simulink model "PMSLM_Close_Loop_MBDL4"  (R2026a)
settings: Solver=FixedStepDiscrete  StopTime=Inf  FixedStep=Ts  EnableMultiTasking=on
values from neighbouring files (symbols this model uses):
  ADC_GainA = 0.01664    [PMSLM_Init_Params_MBDL4.m]
  ADC_GainB = 0.01664    [PMSLM_Init_Params_MBDL4.m]
  ADC_GainC = 0.01664    [PMSLM_Init_Params_MBDL4.m]
  Close_Loop_EN = Simulink.Parameter    [PMSLM_Init_Params_MBDL4.m]
  CPU_Clock = 200e6    (= 200000000)    [PMSLM_Init_Params_MBDL4.m]    (also in init_PMLSM_ThreeLoop_Simple.m)
  delay_N = 50    [PMSLM_Init_Params_MBDL4.m]
  ENCON_Manual = Simulink.Parameter    [PMSLM_Init_Params_MBDL4.m]
  FReset_Manual = Simulink.Parameter    [PMSLM_Init_Params_MBDL4.m]
  GPIO30_PWM_OE_Disable = Simulink.Parameter    [PMSLM_Init_Params_MBDL4.m]
  Grating_Resolution_mm_per_count = 0.0001    [PMSLM_Init_Params_MBDL4.m]
  Hold_Ticks = 30000    [PMSLM_Init_Params_MBDL4.m]
  Id_Init_Step = Id_Init_Target / Ramp_Ticks    (= 5e-05)    [PMSLM_Init_Params_MBDL4.m]
  Id_Init_Target = 0.5    [PMSLM_Init_Params_MBDL4.m]
  Id_Ref_Set = Simulink.Parameter    [PMSLM_Init_Params_MBDL4.m]
  Init_Reset = Simulink.Parameter    [PMSLM_Init_Params_MBDL4.m]
  Init_Start = Simulink.Parameter    [PMSLM_Init_Params_MBDL4.m]
  Iq_fric_run = 0.05    [PMSLM_Init_Params_MBDL4.m]
  Iq_fric_start = 0.40    (= 0.4)    [PMSLM_Init_Params_MBDL4.m]
  Iq_int_limit = 0.10    (= 0.1)    [PMSLM_Init_Params_MBDL4.m]    (also in init_PMLSM_ThreeLoop_Simple.m = 0.5)
  Iq_Test_Mode = Simulink.Parameter    [PMSLM_Init_Params_MBDL4.m]
  Iq_Test_Ref = Simulink.Parameter    [PMSLM_Init_Params_MBDL4.m]
  Kaw_d = Kaw_q    (= 0.2)    [PMSLM_Init_Params_MBDL4.m]    (also in init_PMLSM_ThreeLoop_Simple.m = Tuning_Gains.Kaw_d)
  Kaw_q = 0.2    [PMSLM_Init_Params_MBDL4.m]    (also in init_PMLSM_ThreeLoop_Simple.m = Tuning_Gains.Kaw_q)
  Kaw_s = 0.4    [PMSLM_Init_Params_MBDL4.m]    (also in init_PMLSM_ThreeLoop_Simple.m = Tuning_Gains.Kaw_s)
  Ki_ACR = ACR_Commissioning_Scale*Ki_ACR_Baseline    (= 2962.5)    [PMSLM_Init_Params_MBDL4.m]    (also in init_PMLSM_ThreeLoop_Simple.m = Tuning_Gains.Ki_ACR; init_PMLSM_mil_test_params.m = Kp_ACR*PMLSM_Rs_ohm/PMLSM_Lq_H)
  Ki_ASR = 0.05    [PMSLM_Init_Params_MBDL4.m]    (also in init_PMLSM_ThreeLoop_Simple.m = Tuning_Gains.Ki_ASR)
  Kp_ACR = ACR_Commissioning_Scale*Kp_ACR_Baseline    (= 2.18125)    [PMSLM_Init_Params_MBDL4.m]    (also in init_PMLSM_ThreeLoop_Simple.m = Tuning_Gains.Kp_ACR; init_PMLSM_mil_test_params.m = PMLSM_Lq_H/(4*MIL_AUM3S4_Current_PI_xi^2*MIL_AUM3S4_Current_)
  Kp_ASR = 0.03    [PMSLM_Init_Params_MBDL4.m]    (also in init_PMLSM_ThreeLoop_Simple.m = Tuning_Gains.Kp_ASR)
  Kp_pos = 5    [PMSLM_Init_Params_MBDL4.m]    (also in init_PMLSM_ThreeLoop_Simple.m = Tuning_Gains.Kp_pos)
  OffsetCal_EN = Simulink.Parameter    [PMSLM_Init_Params_MBDL4.m]
  PI_Reset_EN = Simulink.Parameter    [PMSLM_Init_Params_MBDL4.m]
  PMLSM_Ld_H = Ld    (= 0.001745)    [PMSLM_Init_Params_MBDL4.m]    (also in init_PMLSM_ThreeLoop_Simple.m; init_PMLSM_plant_params.m)
  PMLSM_Lq_H = Lq    (= 0.001745)    [PMSLM_Init_Params_MBDL4.m]    (also in init_PMLSM_ThreeLoop_Simple.m; init_PMLSM_plant_params.m)
  PMLSM_psi_f_Wb = flux    (= 0.141)    [PMSLM_Init_Params_MBDL4.m]    (also in init_PMLSM_ThreeLoop_Simple.m; init_PMLSM_plant_params.m)
  Pos_deadband = 0.02    [PMSLM_Init_Params_MBDL4.m]    (also in init_PMLSM_ThreeLoop_Simple.m)
  Pos_Loop_EN = Simulink.Parameter    [PMSLM_Init_Params_MBDL4.m]
  qep_mid_cnt = 2147483648    [PMSLM_Init_Params_MBDL4.m]
  Ramp_Ticks = 10000    [PMSLM_Init_Params_MBDL4.m]
  RELCON_Manual = Simulink.Parameter    [PMSLM_Init_Params_MBDL4.m]
  Speed_loop_Iq_Limit = Iq_Limit    (= 0.3)    [PMSLM_Init_Params_MBDL4.m]    (also in init_PMLSM_ThreeLoop_Simple.m = 1)
  Tau_e_mm = 60    [PMSLM_Init_Params_MBDL4.m]
  theta_align_const = 0    [PMSLM_Init_Params_MBDL4.m]
  Theta_Offset_Fine = Simulink.Parameter    [PMSLM_Init_Params_MBDL4.m]
  Three_Current_Sampling_EN = Simulink.Parameter    [PMSLM_Init_Params_MBDL4.m]
  Ts = 1 / PWM_Freq    (= 0.0001)    [PMSLM_Init_Params_MBDL4.m]    (also in init_PMLSM_ThreeLoop_Simple.m)
  Ts_ACR = 1e-4    (= 0.0001)    [PMSLM_Init_Params_MBDL4.m]    (also in init_PMLSM_ThreeLoop_Simple.m)
  Ts_ASR = 1e-3    (= 0.001)    [PMSLM_Init_Params_MBDL4.m]    (also in init_PMLSM_ThreeLoop_Simple.m)
  Udc = 48    [PMSLM_Init_Params_MBDL4.m]    (also in init_PMLSM_ThreeLoop_Simple.m; init_PMLSM_mil_test_params.m)
  Uq_Zero_EN = 0：q 轴用正常 PI    [PMSLM_Init_Params_MBDL4.m]
  v_ff_eps = 0.5    [PMSLM_Init_Params_MBDL4.m]    (also in init_PMLSM_ThreeLoop_Simple.m)
  V_meas_max = 500    [PMSLM_Init_Params_MBDL4.m]
  v_meas_zero_eps = 0.5    [PMSLM_Init_Params_MBDL4.m]
  v_over_eps = 3    [PMSLM_Init_Params_MBDL4.m]    (also in init_PMLSM_ThreeLoop_Simple.m)
  V_pos_max_mmps = 10    [PMSLM_Init_Params_MBDL4.m]    (also in init_PMLSM_ThreeLoop_Simple.m = 20)
  v_ref_max = 20    [PMSLM_Init_Params_MBDL4.m]    (also in init_PMLSM_ThreeLoop_Simple.m)
  v_ref_set = Simulink.Parameter    [PMSLM_Init_Params_MBDL4.m]
  v_ref_set_step_dn = v_ref_set_rate_dn * Ts    (= 0.005)    [PMSLM_Init_Params_MBDL4.m]    (also in init_PMLSM_ThreeLoop_Simple.m)
  v_ref_set_step_up = v_ref_set_rate_up * Ts    (= 0.005)    [PMSLM_Init_Params_MBDL4.m]    (also in init_PMLSM_ThreeLoop_Simple.m)
  v_ref_zero_eps = 0.2    [PMSLM_Init_Params_MBDL4.m]    (also in init_PMLSM_ThreeLoop_Simple.m = 0)
  v_stick_off = 3.0    (= 3)    [PMSLM_Init_Params_MBDL4.m]
  v_stick_on = 1.0    (= 1)    [PMSLM_Init_Params_MBDL4.m]
  X_max_hard = 500    [PMSLM_Init_Params_MBDL4.m]
  X_max_soft = 470    [PMSLM_Init_Params_MBDL4.m]
  X_min_hard = -500    [PMSLM_Init_Params_MBDL4.m]
  X_min_soft = -470    [PMSLM_Init_Params_MBDL4.m]
  x_ref_mm = Simulink.Parameter    [PMSLM_Init_Params_MBDL4.m]
undefined symbols (not defined in the file or in its folder): bit, Down, GPTRIP1SEL, TZ1, Up
libraries: simulink x11, c2802xlib x6, c2838xlib x6, mcbeeMathTransformLib x2, c280xlib x1, mcbcontrolslib x1, svdschedulerlib x1
(part 1 of 2)
settings Model: ExtModeTrigDuration=8  Creator=lww  LastModifiedBy=lww
settings OptimizationCC: DefaultUnderspecifiedDataType=single  MaxStackSize=1024
settings DebuggingCC: ArtificialAlgebraicLoopMsg=none
settings HardwareCC: ProdBitPerChar=16.0  ProdBitPerInt=16.0  ProdLargestAtomicInteger=Integer  ProdWordSize=16.0  ProdHWDeviceType=Texas Instruments->C2000  HardwareBoardFeatureSet=SoCBlockset
settings ModelReferenceCC: ModelReferenceNumInstancesAllowed=Single
settings RTWCC: SystemTargetFile=ert.tlc  HardwareBoard=TI F2838x  TLCOptions=-aInlineSetEventsForThisBaseRateFcn=TLC_FALSE -aSuppressMultiTaskScheduler=TLC_FALSE -aRateBasedStepFcn=1  Toolchain=Texas Instruments Code Composer Studio - EABI (C2000)  CodeProfilingSaveOptions=MetricsOnly  Description=Embedded Coder
settings ERTTargetCC: ExtModeTransport=4.0  ExtModeAutomaticAllocSize=off  ExtModeStaticAllocSize=10000.0  DynamicArrayContainerType=coder::array  CodeReplacementLibrary=TI C28x  SubcomponentCodeInterfacePackaging=Nonreusable function
settings SimscapeCC: SimscapeNominalValues="[{\"value\":\"1\",\"unit\":\"A\"},{\"value\":\"1\",\"unit\":\"bar\"},{\"value\":\"1\",\"unit\":\"cm^2\"},{\"value\":\"1\",\"unit\":\"cm^3/s\"},{\"value\":\"1\",\"unit\":\"kJ/kg\"},{\"value\":\"1\",\"unit\":\"kW\"},{\"value\":\"1\",\"unit\":\"l\"},{\"value\":\"1\",\"unit\":\"N\"},{\"value\":\"1\",\"unit\":\"N*m\"},{\"value\":\"1\",\"unit\":\"V\"}]"  SimscapeLogType=none  SimscapeLogDataHistory=5000.0

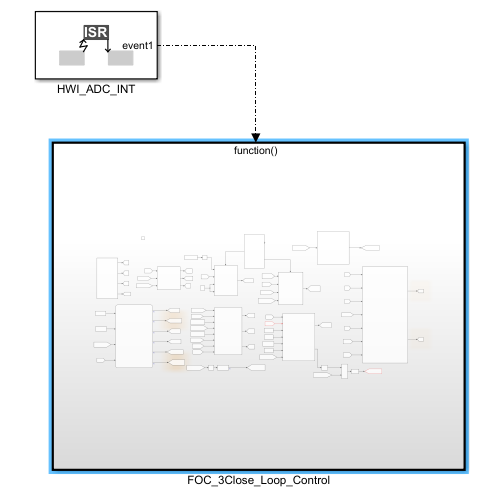
[thumbnail: Simulink's stored preview of the top-level diagram]
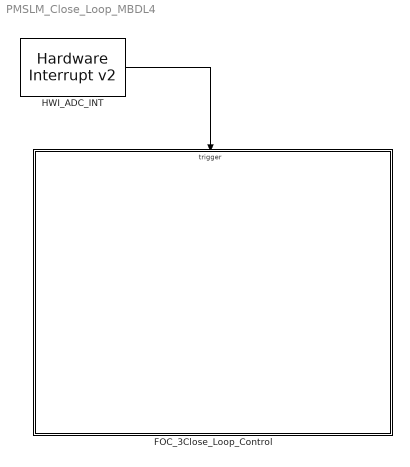
== system PMSLM_Close_Loop_MBDL4 ==
  FOC_3Close_Loop_Control : Subsystem  TreatAsAtomicUnit=on
  HWI_ADC_INT : svdschedulerlib/Hardware Interrupt v2  ISRGroup=ADC - Analog to Digital Converter  ISRName=ADCA1_INT  ISRNumber=32  NumEventsToServe=1  EventsList={'on','EOC event','1';'off','Overflow event','2';'off','Custom event','3'}  SelectedEvents={'event1'}  TaskPriority=30  DisablePreemption=on  ClearInterruptFlagsAtEndOfEvent=on  InterruptDefinitionFile=$(TARGET_ROOT)/registry/interrupts/TIF2838x_c28xCPU1_interrupts.xml  HardwareBoard=TI F2838x  EnableSimPort=off
  wires:
  HWI_ADC_INT/1 -> FOC_3Close_Loop_Control/Trigger

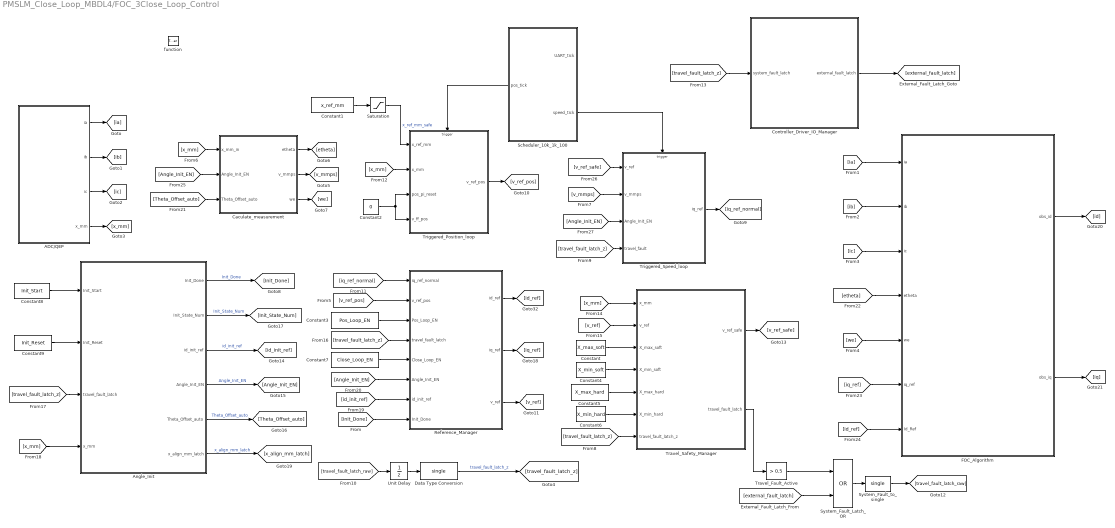
== system PMSLM_Close_Loop_MBDL4/FOC_3Close_Loop_Control ==
  function : TriggerPort  TriggerType=function-call  VariantControl=(inherit)
  ADC/QEP : Subsystem
  Angle_Init : Stateflow chart  TreatAsAtomicUnit=on
  Caculate_measurement : Subsystem
  Constant : Constant  Value=X_max_soft
  Constant1 : Constant  Value=x_ref_mm
  Constant2 : Constant  Value=0
  Constant3 : Constant  Value=Pos_Loop_EN
  Constant4 : Constant  Value=X_min_soft
  Constant5 : Constant  Value=X_max_hard
  Constant6 : Constant  Value=X_min_hard
  Constant7 : Constant  Value=Close_Loop_EN
  Constant8 : Constant  Value=Init_Start
  Constant9 : Constant  Value=Init_Reset
  Controller_Driver_IO_Manager : Subsystem
  Data Type Conversion : DataTypeConversion  OutDataTypeStr=single  SaturateOnIntegerOverflow=off  RndMeth=Floor
  FOC_Algorithm : Subsystem
  Reference_Manager : Subsystem
  Saturation : Saturate  UpperLimit=X_max_soft  LowerLimit=X_min_soft
  Scheduler_10k_1k_100 : Subsystem
      settings: PortSchema="{\"entries\":[{\"content\":{\"sides\":[{\"content\":{\"connectorIds\":[\"Out3\"]},\"type\":\"ConnectorPlacement.EquallySpacedRectSide\",\"uuid\":\"7a2cd2ad-1b6d-4ced-b4c0-dea2e76e4441\"},{\"content\":{\"connectorIds\":[\"Out1\",\"Out2\"],\"side\":\"RIGHT\"},\"type\":\"ConnectorPlacement.EquallySpacedRectSide\",\"uuid\":\"f7db3b94-1126-4089-83bd-8e57d20e6fd7\"},{\"content\":{\"side\":\"TOP\"},\"type\":\"ConnectorPlacement.EquallySpacedRectSide\",\"uuid\":\"9153f6b5-22af-48be-92c0-68be43f93648\"}]},\"type\":\"ConnectorPlacement.EquallySpacedConnector\",\"uuid\":\"029fb485-bddc-4cd2-9c64-7547c8dffd2b\"}],\"packageUris\":[\"http://schema.mathworks.com/mf0/Connector/R2020b\"],\"version\":\"1.0\"}"
  System_Fault_Latch_OR : Logic  Operator=OR
  System_Fault_to_single : DataTypeConversion  OutDataTypeStr=single
  Travel_Fault_Active : simulink/Logic and Bit Operations/Compare To Constant  relop=>  const=0.5  OutDataTypeStr=boolean
  Travel_Safety_Manager : MATLAB Function  TreatAsAtomicUnit=on
  Triggered_Position_loop : Subsystem  TreatAsAtomicUnit=on
  Triggered_Speed_loop : Subsystem  TreatAsAtomicUnit=on
  Unit Delay : UnitDelay  SampleTime=-1
  wires:
  [iq_ref_normal] -> Reference_Manager/1(iq_ref_normal)
  ADC/QEP/3(ic) -> [ic]
  Caculate_measurement/2(v_mmps) -> [v_mmps]
  [v_mmps] -> Triggered_Speed_loop/2(v_mmps)
  Caculate_measurement/1(etheta) -> [etheta]
  Reference_Manager/1(id_ref) -> [id_ref]
  Scheduler_10k_1k_100/2(speed_tick) -> Triggered_Speed_loop/Trigger
  [v_ref_safe] -> Triggered_Speed_loop/1(v_ref)
  Reference_Manager/2(iq_ref) -> [iq_ref]
  ADC/QEP/1(ia) -> [ia]
  Triggered_Speed_loop/1(iq_ref) -> [iq_ref_normal]
  ADC/QEP/2(ib) -> [ib]
  [ia] -> FOC_Algorithm/1(ia)
  [ib] -> FOC_Algorithm/2(ib)
  [ic] -> FOC_Algorithm/3(ic)
  [etheta] -> FOC_Algorithm/4(etheta)
  [we] -> FOC_Algorithm/5(we)
  [iq_ref] -> FOC_Algorithm/6(iq_ref)
  [x_mm] -> Triggered_Position_loop/2(x_mm)
  Constant2/1 -> Triggered_Position_loop/3(pos_pi_reset), Triggered_Position_loop/4(v_ff_pos)
  Triggered_Position_loop/1(v_ref_pos) -> [v_ref_pos]
  [v_ref_pos] -> Reference_Manager/2(v_ref_pos)
  Constant3/1 -> Reference_Manager/3(Pos_Loop_EN)
  ADC/QEP/4(x_mm) -> [x_mm]
  Caculate_measurement/3(we) -> [we]
  [x_mm] -> Caculate_measurement/1(x_mm_in)
  Reference_Manager/3(v_ref) -> [v_ref]
  Constant1/1 -> Saturation/1
  Saturation/1 -> Triggered_Position_loop/1(x_ref_mm)  "x_ref_mm_safe"
  [travel_fault_latch_z] -> Triggered_Speed_loop/4(travel_fault)
  [travel_fault_latch_raw] -> Unit Delay/1
  [id_ref] -> FOC_Algorithm/7(Id_Ref)
  [travel_fault_latch_z] -> Controller_Driver_IO_Manager/1(system_fault_latch)
  [x_mm] -> Travel_Safety_Manager/1(x_mm)
  [v_ref] -> Travel_Safety_Manager/2(v_ref)
  Constant/1 -> Travel_Safety_Manager/3(X_max_soft)
  Constant4/1 -> Travel_Safety_Manager/4(X_min_soft)
  Constant5/1 -> Travel_Safety_Manager/5(X_max_hard)
  Constant6/1 -> Travel_Safety_Manager/6(X_min_hard)
  Travel_Safety_Manager/1(v_ref_safe) -> [v_ref_safe]
  [travel_fault_latch_z] -> Travel_Safety_Manager/7(travel_fault_latch_z)
  Unit Delay/1 -> Data Type Conversion/1
  Data Type Conversion/1 -> [travel_fault_latch_z]  "travel_fault_latch_z"
  [travel_fault_latch_z] -> Reference_Manager/4(travel_fault_latch)
  Constant7/1 -> Reference_Manager/5(Close_Loop_EN)
  Constant8/1 -> Angle_Init/1(Init_Start)
  Constant9/1 -> Angle_Init/2(Init_Reset)
  [travel_fault_latch_z] -> Angle_Init/3(travel_fault_latch)
  Angle_Init/1(Init_Done) -> [Init_Done]  "Init_Done"
  [Init_Done] -> Reference_Manager/8(Init_Done)
  [x_mm] -> Angle_Init/4(x_mm)
  Angle_Init/3(id_init_ref) -> [id_init_ref]  "id_init_ref"
  [id_init_ref] -> Reference_Manager/7(id_init_ref)
  Angle_Init/4(Angle_Init_EN) -> [Angle_Init_EN]  "Angle_Init_EN"
  [Angle_Init_EN] -> Reference_Manager/6(Angle_Init_EN)
  Angle_Init/5(Theta_Offset_auto) -> [Theta_Offset_auto]  "Theta_Offset_auto"
  [Theta_Offset_auto] -> Caculate_measurement/3(Theta_Offset_auto)
  [Angle_Init_EN] -> Caculate_measurement/2(Angle_Init_EN)
  Angle_Init/2(Init_State_Num) -> [Init_State_Num]  "Init_State_Num"
  [Angle_Init_EN] -> Triggered_Speed_loop/3(Angle_Init_EN)
  Angle_Init/6(x_align_mm_latch) -> [x_align_mm_latch]  "x_align_mm_latch"
  FOC_Algorithm/1(obs_id) -> [id]
  FOC_Algorithm/2(obs_iq) -> [iq]
  Scheduler_10k_1k_100/3(pos_tick) -> Triggered_Position_loop/Trigger
  Travel_Safety_Manager/2(travel_fault_latch) -> Travel_Fault_Active/1
  Travel_Fault_Active/1 -> System_Fault_Latch_OR/1
  System_Fault_Latch_OR/1 -> System_Fault_to_single/1
  System_Fault_to_single/1 -> [travel_fault_latch_raw]
  Controller_Driver_IO_Manager/1(external_fault_latch) -> [external_fault_latch]
  [external_fault_latch] -> System_Fault_Latch_OR/2

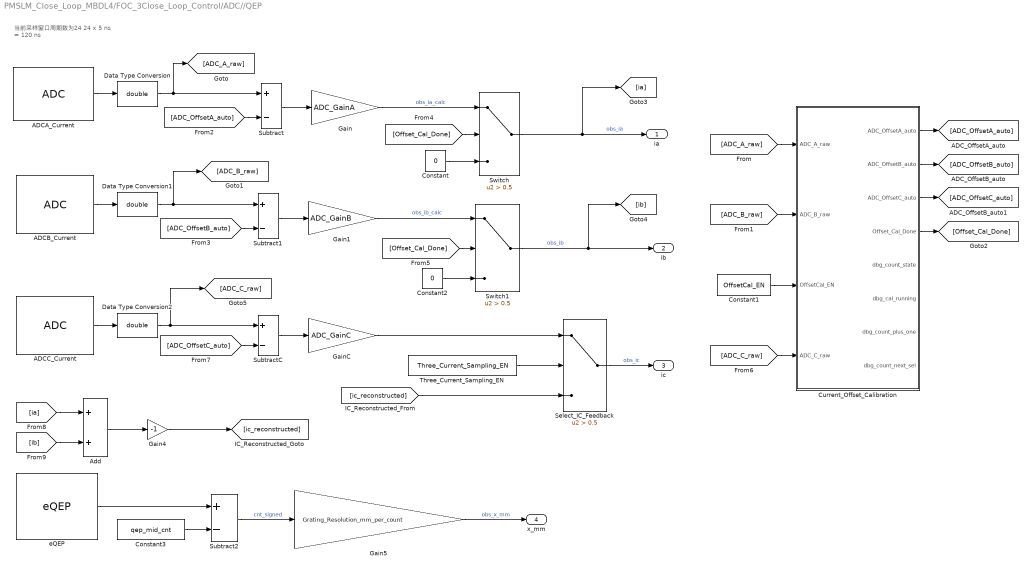
== system PMSLM_Close_Loop_MBDL4/FOC_3Close_Loop_Control/ADC//QEP ==
  note: 当前采样窗口周期数为24
      | 24 x 5 ns = 120 ns
  ADCA_Current : c2802xlib/ADC  blkParamProc=C2000_Type4  ADCModule=A  samplingMode=Single sample mode  ADCResolution=12-bit (Single-ended input)  ADC29xResolution=12-bit  ADCMode=Single-ended input  useSOC1=SOC0  useSOC2=SOC0_SOC1  SOCAcquisitionWindow=24  SOCTriggerSource=ePWM1_ADCSOCA  SOCInterruptTrigger=No ADCINT  Ts=-1  dType=uint16  postInterrupt=on  interruptSel=ADCINT1  ADCINTContinuous=off  endma=off  chdma=1  conv1=ADCINA0  conv2=ADCINA0 and ADCINB0  conv1_Type4=ADCIN0  conv2_Type4=ADCIN0 and ADCIN1
      settings: LibrarySourceBlock=c2838xlib/ADC
  ADCB_Current : c2802xlib/ADC  blkParamProc=C2000_Type4  ADCModule=B  samplingMode=Single sample mode  ADCResolution=12-bit (Single-ended input)  ADC29xResolution=12-bit  ADCMode=Single-ended input  useSOC1=SOC0  useSOC2=SOC0_SOC1  SOCAcquisitionWindow=24  SOCTriggerSource=ePWM1_ADCSOCA  SOCInterruptTrigger=No ADCINT  Ts=-1  dType=uint16  postInterrupt=off  interruptSel=ADCINT1  ADCINTContinuous=on  endma=off  chdma=1  conv1=ADCINA0  conv2=ADCINA0 and ADCINB0  conv1_Type4=ADCIN0  conv2_Type4=ADCIN0 and ADCIN1
      settings: LibrarySourceBlock=c2838xlib/ADC
  ADCC_Current : c2802xlib/ADC  blkParamProc=C2000_Type4  ADCModule=C  samplingMode=Single sample mode  ADCResolution=12-bit (Single-ended input)  ADC29xResolution=12-bit  ADCMode=Single-ended input  useSOC1=SOC0  useSOC2=SOC0_SOC1  SOCAcquisitionWindow=24  SOCTriggerSource=ePWM1_ADCSOCA  SOCInterruptTrigger=No ADCINT  Ts=-1  dType=uint16  postInterrupt=off  interruptSel=ADCINT1  ADCINTContinuous=on  endma=off  chdma=1  conv1=ADCINA0  conv2=ADCINA0 and ADCINB0  conv1_Type4=ADCIN2  conv2_Type4=ADCIN0 and ADCIN1
      settings: LibrarySourceBlock=c2838xlib/ADC
  Add : Sum
  Constant : Constant  Value=0  OutDataTypeStr=double
  Constant1 : Constant  Value=OffsetCal_EN
  Constant2 : Constant  Value=0  OutDataTypeStr=double
  Constant3 : Constant  Value=qep_mid_cnt
  Current_Offset_Calibration : Subsystem
  Data Type Conversion : DataTypeConversion  OutDataTypeStr=double  SaturateOnIntegerOverflow=off  RndMeth=Floor
  Data Type Conversion1 : DataTypeConversion  OutDataTypeStr=double  SaturateOnIntegerOverflow=off  RndMeth=Floor
  Data Type Conversion2 : DataTypeConversion  OutDataTypeStr=double
  Gain : Gain  Gain=ADC_GainA
  Gain1 : Gain  Gain=ADC_GainB
  Gain4 : Gain  Gain=-1  OutDataTypeStr=double
  Gain5 : Gain  Gain=Grating_Resolution_mm_per_count
  GainC : Gain  Gain=ADC_GainC
  Select_IC_Feedback : Switch  Criteria=u2 > Threshold  Threshold=0.5  OutDataTypeStr=double
  Subtract : Sum  Inputs=+-
  Subtract1 : Sum  Inputs=+-
  Subtract2 : Sum  Inputs=+-
  SubtractC : Sum  Inputs=+-
  Switch : Switch  Criteria=u2 > Threshold  Threshold=0.5  OutDataTypeStr=double  SaturateOnIntegerOverflow=off  InputSameDT=off
  Switch1 : Switch  Criteria=u2 > Threshold  Threshold=0.5  OutDataTypeStr=double  SaturateOnIntegerOverflow=off  InputSameDT=off
  Three_Current_Sampling_EN : Constant  Value=Three_Current_Sampling_EN
  eQEP : c280xlib/eQEP  useModule=eQEP1  pcInputmode=Quadrature-count  externalClockrate=2x resolution: Count the rising/falling edge  swapPolarityselection=Clockwise  qdfOutputport=off  qapPolarityselection=off  qbpPolarityselection=off  qipPolarityselection=off  qspPolarityselection=off  igatePolarityselection=off  sampleTime=-1  pcOutputport=on  pcMaximumvalue=4294967295  indexInitializationcheck=off  indexInitializationevent=Rising edge  strobeInitializationcheck=off  strobeInitializationevent=Rising edge  softwareInitializationcheck=off  softwareInitializationsource=Set to init value at start up  softwareInitializationmode=on  pcInitialvalue=qep_mid_cnt  pcResetmode=Reset on an index event  ieloutputport=off  indexEventlatch=Rising edge  seloutputport=off  strobeEventlatch=Rising edge  pcefOutputport=off  enableEqepcapture=off  qctmrOutputport=off  qcprdOutputport=off  captureTimerprescaler=128  upEventprescaler=128  overflowErrorflag=off  directionErrorflag=off  captureTimerposition=On position counter read  unitTimerperiod=100000000  captureTimerlatch=off  capturePeriodlatch=off  positionCounterlatch=off  soenPolarityselection=off  spselPolarityselection=Index pin is used for sync output  compareValuesource=Specify via dialog  shadowMode=Load on QPOSCNT=0  compareValue=4294967295  syncOutputwidth=1  polaritySyncoutput=Active high  watchdogEnable=off  watchdogTimer=65535  outport1Datatype=auto  outport2Datatype=auto  outport3Datatype=auto  outport4Datatype=auto  outport5Datatype=auto  outport6Datatype=auto  outport7Datatype=auto  outport8Datatype=auto  outport9Datatype=auto  outport10Datatype=auto  outport11Datatype=auto  outport12Datatype=auto  eqepinterrupt_pce=off  eqepinterrupt_qpe=off  eqepinterrupt_qdc=off  eqepinterrupt_wto=off  eqepinterrupt_pcu=off  eqepinterrupt_pco=off  eqepinterrupt_pcr=off  eqepinterrupt_pcm=off  eqepinterrupt_sel=off  eqepinterrupt_iel=off  eqepinterrupt_uto=off  pheOutputport=off  watchdogOutputport=off  outport13Datatype=auto  outport14Datatype=auto
      settings: LibrarySourceBlock=c2838xlib/eQEP
  ia : Outport
  ib : Outport  Port=2
  ic : Outport  Port=3
  x_mm : Outport  Port=4
  wires:
  ADCA_Current/1 -> Data Type Conversion/1
  Data Type Conversion/1 -> [ADC_A_raw], Subtract/1
  [ADC_OffsetA_auto] -> Subtract/2
  Subtract/1 -> Gain/1
  Gain/1 -> Switch/1  "obs_ia_calc"
  [Offset_Cal_Done] -> Switch/2
  Constant/1 -> Switch/3
  Switch/1 -> ia/1, [ia]  "obs_ia"
  ADCB_Current/1 -> Data Type Conversion1/1
  Data Type Conversion1/1 -> [ADC_B_raw], Subtract1/1
  [ADC_OffsetB_auto] -> Subtract1/2
  Subtract1/1 -> Gain1/1
  Gain1/1 -> Switch1/1  "obs_ib_calc"
  [Offset_Cal_Done] -> Switch1/2
  Constant2/1 -> Switch1/3
  Switch1/1 -> [ib], ib/1  "obs_ib"
  ADCC_Current/1 -> Data Type Conversion2/1
  Data Type Conversion2/1 -> [ADC_C_raw], SubtractC/1
  [ADC_OffsetC_auto] -> SubtractC/2
  SubtractC/1 -> GainC/1
  GainC/1 -> Select_IC_Feedback/1
  Three_Current_Sampling_EN/1 -> Select_IC_Feedback/2
  Select_IC_Feedback/1 -> ic/1  "obs_ic"
  [ia] -> Add/1
  [ib] -> Add/2
  Add/1 -> Gain4/1
  Gain4/1 -> [ic_reconstructed]
  eQEP/1 -> Subtract2/1
  Constant3/1 -> Subtract2/2
  Subtract2/1 -> Gain5/1  "cnt_signed"
  Gain5/1 -> x_mm/1  "obs_x_mm"
  [ADC_A_raw] -> Current_Offset_Calibration/1(ADC_A_raw)
  [ADC_B_raw] -> Current_Offset_Calibration/2(ADC_B_raw)
  Constant1/1 -> Current_Offset_Calibration/3(OffsetCal_EN)
  Current_Offset_Calibration/1(ADC_OffsetA_auto) -> [ADC_OffsetA_auto]
  Current_Offset_Calibration/2(ADC_OffsetB_auto) -> [ADC_OffsetB_auto]
  Current_Offset_Calibration/4(Offset_Cal_Done) -> [Offset_Cal_Done]
  [ic_reconstructed] -> Select_IC_Feedback/3
  [ADC_C_raw] -> Current_Offset_Calibration/4(ADC_C_raw)
  Current_Offset_Calibration/3(ADC_OffsetC_auto) -> [ADC_OffsetC_auto]

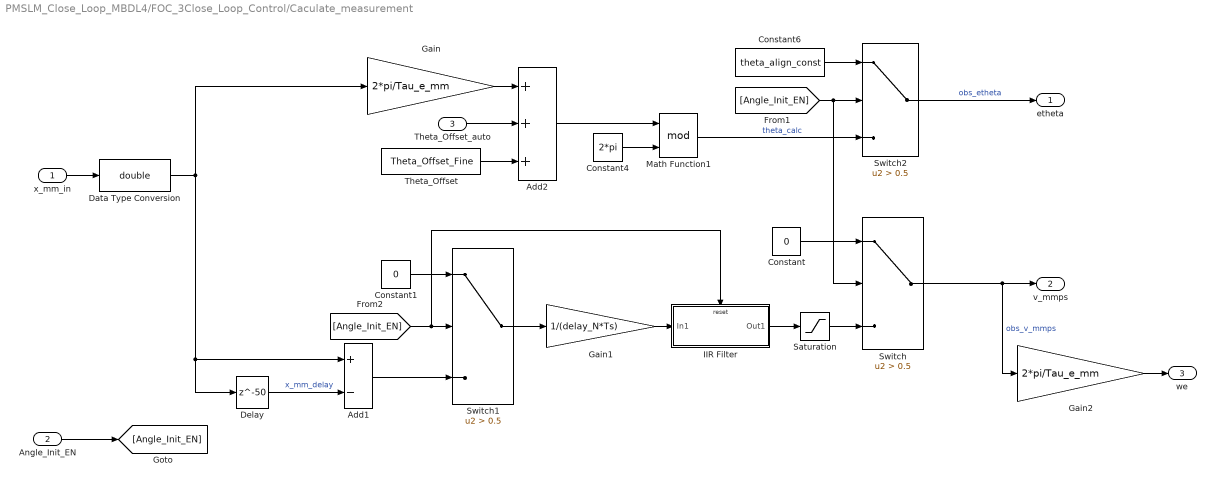
== system PMSLM_Close_Loop_MBDL4/FOC_3Close_Loop_Control/Caculate_measurement ==
  x_mm_in : Inport
  Angle_Init_EN : Inport  Port=2
  Theta_Offset_auto : Inport  Port=3
  Add1 : Sum  Inputs=+-
  Add2 : Sum  Inputs=+++
  Constant : Constant  Value=0
  Constant1 : Constant  Value=0
  Constant4 : Constant  Value=2*pi
  Constant6 : Constant  Value=theta_align_const
  Data Type Conversion : DataTypeConversion  OutDataTypeStr=double  SaturateOnIntegerOverflow=off  RndMeth=Floor
  Delay : Delay  DelayLength=50
  Gain : Gain  Gain=2*pi/Tau_e_mm
  Gain1 : Gain  Gain=1/(delay_N*Ts)
  Gain2 : Gain  Gain=2*pi/Tau_e_mm
  IIR Filter : Subsystem  TreatAsAtomicUnit=on
  Math Function1 : Math  Operator=mod
  Saturation : Saturate  UpperLimit=V_meas_max  LowerLimit=-V_meas_max
  Switch : Switch  Criteria=u2 > Threshold  Threshold=0.5  SaturateOnIntegerOverflow=off  InputSameDT=off
  Switch1 : Switch  Criteria=u2 > Threshold  Threshold=0.5  SaturateOnIntegerOverflow=off  InputSameDT=off
  Switch2 : Switch  Criteria=u2 > Threshold  Threshold=0.5  SaturateOnIntegerOverflow=off  InputSameDT=off
  Theta_Offset : Constant  Value=Theta_Offset_Fine
  etheta : Outport
  v_mmps : Outport  Port=2
  we : Outport  Port=3
  wires:
  x_mm_in/1 -> Data Type Conversion/1
  Delay/1 -> Add1/2  "x_mm_delay"
  Gain/1 -> Add2/1
  Add2/1 -> Math Function1/1
  Constant4/1 -> Math Function1/2
  Data Type Conversion/1 -> Delay/1, Add1/1, Gain/1
  Switch/1 -> Gain2/1, v_mmps/1  "obs_v_mmps"
  Constant/1 -> Switch/1
  Constant1/1 -> Switch1/1
  Switch1/1 -> Gain1/1
  Add1/1 -> Switch1/3
  IIR Filter/1(Out1) -> Saturation/1
  Gain1/1 -> IIR Filter/1(In1)
  Saturation/1 -> Switch/3
  [Angle_Init_EN] -> Switch2/2, Switch/2
  Math Function1/1 -> Switch2/3  "theta_calc"
  Switch2/1 -> etheta/1  "obs_etheta"
  Angle_Init_EN/1 -> [Angle_Init_EN]
  Constant6/1 -> Switch2/1
  Gain2/1 -> we/1
  [Angle_Init_EN] -> Switch1/2, IIR Filter/Reset
  Theta_Offset/1 -> Add2/3
  Theta_Offset_auto/1 -> Add2/2

== system PMSLM_Close_Loop_MBDL4/FOC_3Close_Loop_Control/Controller_Driver_IO_Manager ==
  note: GPIO30 only controls the PWM level-shifter active-low /OE.
      | RELCON, ENCON and F_Reset use independent GPIO outputs.
      | System fault: TZ1/TZ2 hardware trip + software latch; GPIO30=1 and RELCON/ENCON=0.
  note: GPIO67: ERRI; GPIO68: ERRU (active-low inputs)
  note: GPIO62: RELCON
  note: GPIO63: ENCON
  note: GPIO66: F_Reset
  note: GPIO30: PWM level-shifter /OE (1=disable, 0=enable)
  system_fault_latch : Inport
  Constant : Constant  Value=RELCON_Manual
  Constant2 : Constant  Value=GPIO30_PWM_OE_Disable
  Constant4 : Constant  Value=ENCON_Manual
  Constant5 : Constant  Value=FReset_Manual
  ENCON_Safe_Enable : Logic
  External_Fault_Latch : Subsystem
  GPIO30_PWM_OE : c2838xlib/Digital Output  GPIO_Number=GPIO24~GPIO31  GPIO_Bit0=off  GPIO_BIT0_Toggle=off  GPIO_Bit1=off  GPIO_BIT1_Toggle=off  GPIO_Bit2=off  GPIO_BIT2_Toggle=off  GPIO_Bit3=off  GPIO_BIT3_Toggle=off  GPIO_Bit4=off  GPIO_BIT4_Toggle=off  GPIO_Bit5=off  GPIO_BIT5_Toggle=off  GPIO_Bit6=on  GPIO_BIT6_Toggle=off  GPIO_Bit7=off  GPIO_BIT7_Toggle=off
  GPIO62_RELCON : c2838xlib/Digital Output  GPIO_Number=GPIO56~GPIO63  GPIO_Bit0=off  GPIO_BIT0_Toggle=off  GPIO_Bit1=off  GPIO_BIT1_Toggle=off  GPIO_Bit2=off  GPIO_BIT2_Toggle=off  GPIO_Bit3=off  GPIO_BIT3_Toggle=off  GPIO_Bit4=off  GPIO_BIT4_Toggle=off  GPIO_Bit5=off  GPIO_BIT5_Toggle=off  GPIO_Bit6=on  GPIO_BIT6_Toggle=off  GPIO_Bit7=off  GPIO_BIT7_Toggle=off
  GPIO63_ENCON : c2838xlib/Digital Output  GPIO_Number=GPIO56~GPIO63  GPIO_Bit0=off  GPIO_BIT0_Toggle=off  GPIO_Bit1=off  GPIO_BIT1_Toggle=off  GPIO_Bit2=off  GPIO_BIT2_Toggle=off  GPIO_Bit3=off  GPIO_BIT3_Toggle=off  GPIO_Bit4=off  GPIO_BIT4_Toggle=off  GPIO_Bit5=off  GPIO_BIT5_Toggle=off  GPIO_Bit6=off  GPIO_BIT6_Toggle=off  GPIO_Bit7=on  GPIO_BIT7_Toggle=off
  GPIO66_F_Reset : c2838xlib/Digital Output  GPIO_Number=GPIO64~GPIO71  GPIO_Bit0=off  GPIO_BIT0_Toggle=off  GPIO_Bit1=off  GPIO_BIT1_Toggle=off  GPIO_Bit2=on  GPIO_BIT2_Toggle=off  GPIO_Bit3=off  GPIO_BIT3_Toggle=off  GPIO_Bit4=off  GPIO_BIT4_Toggle=off  GPIO_Bit5=off  GPIO_BIT5_Toggle=off  GPIO_Bit6=off  GPIO_BIT6_Toggle=off  GPIO_Bit7=off  GPIO_BIT7_Toggle=off
  GPIO67_ERRI : c2838xlib/Digital Input  GPIO_Number=GPIO64~GPIO71  GPIO_Bit0=off  GPIO_Bit1=off  GPIO_Bit2=off  GPIO_Bit3=on  GPIO_Bit4=off  GPIO_Bit5=off  GPIO_Bit6=off  GPIO_Bit7=off  sampleTime=-1  dataType=boolean  GPIO_Bit0_Qualification=Sync to SYSCLKOUT  GPIO_Bit1_Qualification=Sync to SYSCLKOUT  GPIO_Bit2_Qualification=Sync to SYSCLKOUT  GPIO_Bit3_Qualification=Sync to SYSCLKOUT  GPIO_Bit4_Qualification=Sync to SYSCLKOUT  GPIO_Bit5_Qualification=Sync to SYSCLKOUT  GPIO_Bit6_Qualification=Sync to SYSCLKOUT  GPIO_Bit7_Qualification=Sync to SYSCLKOUT  Qualification_Period=-1
  GPIO68_ERRU : c2838xlib/Digital Input  GPIO_Number=GPIO64~GPIO71  GPIO_Bit0=off  GPIO_Bit1=off  GPIO_Bit2=off  GPIO_Bit3=off  GPIO_Bit4=on  GPIO_Bit5=off  GPIO_Bit6=off  GPIO_Bit7=off  sampleTime=-1  dataType=boolean  GPIO_Bit0_Qualification=Sync to SYSCLKOUT  GPIO_Bit1_Qualification=Sync to SYSCLKOUT  GPIO_Bit2_Qualification=Sync to SYSCLKOUT  GPIO_Bit3_Qualification=Sync to SYSCLKOUT  GPIO_Bit4_Qualification=Sync to SYSCLKOUT  GPIO_Bit5_Qualification=Sync to SYSCLKOUT  GPIO_Bit6_Qualification=Sync to SYSCLKOUT  GPIO_Bit7_Qualification=Sync to SYSCLKOUT  Qualification_Period=-1
  Logical Operator : Logic  Operator=OR  AllPortsSameDT=off  OutDataTypeStr=boolean
  RELCON_Safe_Enable : Logic
  System_Fault_Active : simulink/Logic and Bit Operations/Compare To Constant  relop=>  const=0.5  OutDataTypeStr=boolean
  System_Fault_Not : Logic  Operator=NOT  Inputs=1
  external_fault_latch : Outport  OutDataTypeStr=boolean  PortDimensions=1
  wires:
  Constant2/1 -> Logical Operator/1
  Logical Operator/1 -> GPIO30_PWM_OE/1
  system_fault_latch/1 -> System_Fault_Active/1
  System_Fault_Active/1 -> Logical Operator/2, System_Fault_Not/1
  System_Fault_Not/1 -> [drive_safe]
  GPIO67_ERRI/1 -> [ERRI_raw]
  [ERRI_raw] -> External_Fault_Latch/1(ERRI_raw)
  GPIO68_ERRU/1 -> [ERRU_raw]
  [ERRU_raw] -> External_Fault_Latch/2(ERRU_raw)
  Constant/1 -> RELCON_Safe_Enable/1  "obs_RELCON"
  RELCON_Safe_Enable/1 -> GPIO62_RELCON/1
  Constant4/1 -> ENCON_Safe_Enable/1
  [drive_safe] -> ENCON_Safe_Enable/2
  ENCON_Safe_Enable/1 -> GPIO63_ENCON/1
  Constant5/1 -> GPIO66_F_Reset/1
  External_Fault_Latch/1(external_fault_latch) -> external_fault_latch/1
  [drive_safe] -> RELCON_Safe_Enable/2

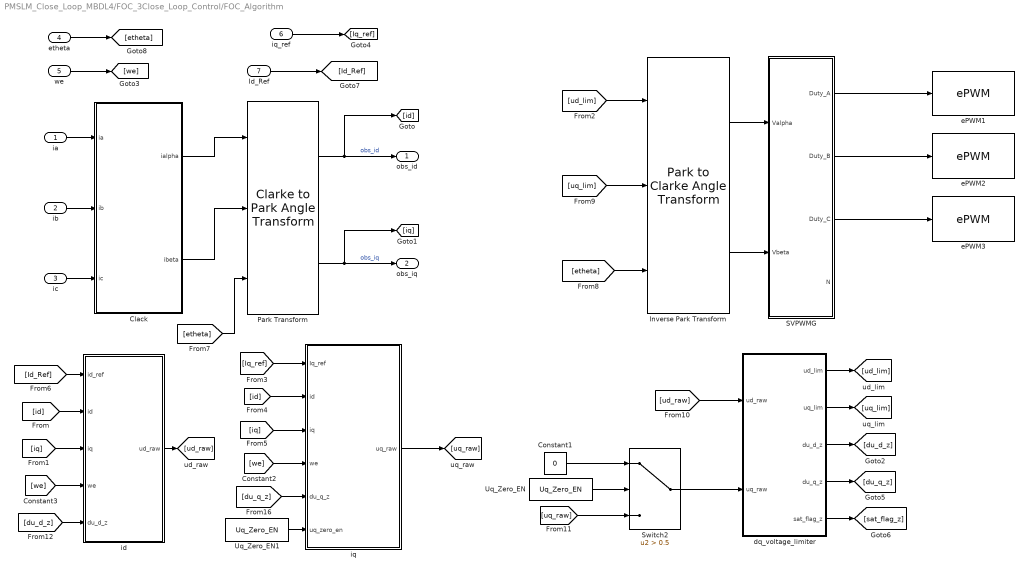
== system PMSLM_Close_Loop_MBDL4/FOC_3Close_Loop_Control/FOC_Algorithm ==
  ia : Inport
  ib : Inport  Port=2
  ic : Inport  Port=3
  etheta : Inport  Port=4
  we : Inport  Port=5
  iq_ref : Inport  Port=6
  Id_Ref : Inport  Port=7
  Clack : Subsystem  TreatAsAtomicUnit=on  RTWFcnName=Clack_Fun
      settings: RTWFcnNameOpts=User specified
  Constant1 : Constant  Value=0  OutDataTypeStr=double
  Inverse Park Transform : mcbeeMathTransformLib/Park to Clarke Angle Transform  AxisAlignment=D-axis  UseWithEmbedded=on  PhaseInput=Two inputs  ThetaInput=Electrical position  AngleInput=Radians  N_points=1024
      settings: LibrarySourceBlock=mcbhdllib/Controls/Math Transforms/Inverse Park Transform
  Park Transform : mcbeeMathTransformLib/Clarke to Park Angle Transform  AxisAlignment=D-axis  UseWithEmbedded=on  PhaseInput=Two inputs  ThetaInput=Electrical position  AngleInput=Radians  N_points=1024
      settings: LibrarySourceBlock=mcblib/Controls/Math Transforms/Park Transform
  SVPWMG : Subsystem  TreatAsAtomicUnit=on  RTWFcnName=SVPWM_Gen_Fun
      settings: RTWFcnNameOpts=User specified
  Switch2 : Switch  Criteria=u2 > Threshold  Threshold=0.5  SaturateOnIntegerOverflow=off  InputSameDT=off
  Uq_Zero_EN : Constant  Value=Uq_Zero_EN
  Uq_Zero_EN1 : Constant  Value=Uq_Zero_EN
  dq_voltage_limiter : Subsystem
  ePWM1 : c2802xlib/ePWM  PwmType=C2000_Type4_F2838x  useModule=ePWM1  ePWMxLINKTBPRD=Not Linked  periodUnits=Clock cycles  timerSource=Specify via dialog  timerPeriod_clk=PWM_Period  timerPeriod_sec=0.0001  tbshadow=Counter equals to zero  countingMode=Up-Down  phaseActiveEnable=Disable  phaseDirection=Count down after sync  phaseActive=0  synchronizationEnable=off  dcaevt1Sync=off  dcbevt1Sync=off  synchronizationOption=Disable  dcbevt1SyncOut=off  dcaevt1SyncOut=off  cmpdSyncOut=off  cmpcSyncOut=off  cmpbSyncOut=off  zeroSyncOut=off  swfSyncOut=off  perSynchronizationOption=Counter equals to period (CTR=PRD)  clockPrescale=1  HSclockPrescale=1  enswap=off  ePWMxAStatus=on  ePWMxAactionLogic1=Do nothing  ePWMxAactionLogic2=Do nothing  ePWMxAactionLogic3=Clear  ePWMxAactionLogic4=Set  ePWMxAactionLogic5=Do nothing  ePWMxAactionLogic6=Do nothing  ePWMxACSFenable=off  ePWMxACSFvalue=Forcing disable  ePWMxASFreload=Zero  ePWMxBStatus=on  ePWMxBactionLogic1=Set  ePWMxBactionLogic2=Clear  ePWMxBactionLogic3=Do nothing  ePWMxBactionLogic4=Do nothing  ePWMxBactionLogic5=Clear  ePWMxBactionLogic6=Set  ePWMxBCSFenable=off  ePWMxBCSFvalue=Forcing disable  ePWMxBSFreload=Zero  ePWNxBOutWay=off  ePWMxLINKCMPA=Not Linked  CMPAUnits=Clock cycles  CMPASource=Input port  CMPAValue_per=50  CMPAValue_clk=32000  enCMPAshadow=Counter equals to zero (CTR=Zero)  ePWMxLINKCMPB=Not Linked  CMPBUnits=Clock cycles  CMPBSource=Specify via dialog  CMPBValue_per=50  CMPBValue_clk=32000  enCMPBshadow=Counter equals to zero (CTR=Zero)  ePWMxLINKCMPC=Not Linked  CMPCUnits=Clock cycles  CMPCSource=Specify via dialog  CMPCValue_per=50  CMPCValue_clk=32000  enCMPCshadow=Counter equals to zero (CTR=Zero)  ePWMxLINKCMPD=Not Linked  CMPDUnits=Clock cycles  CMPDSource=Specify via dialog  CMPDValue_per=50  CMPDValue_clk=32000  enCMPDshadow=Counter equals to zero (CTR=Zero)  enableDBePWMxA=on  enableDBePWMxB=on  enhalfcycle=off  DBpolarity=Active high complementary (AHC)  DBedgeDelay=Positive  DBSource_ePWMxA=ePWMxA  DBSource_ePWMxB=ePWMxA  DBPeriodUnits=Clock cycles  DBperiodSource=Specify via dialog  REDperiod=PWM_DeadTime_Count  FEDperiod=PWM_DeadTime_Count  REDperiod_sec=0  FEDperiod_sec=0  LoadModeDBRED=Immediate without using shadow  LoadModeDBFED=Immediate without using shadow  adcstartModuleA=on  adcrequestEventA=First event  adcstartEventA=Counter equals to period (CTR=PRD)  adcstartEventA_type2=Counter equals to period (CTR=PRD)  adcstartModuleB=off  adcrequestEventB=First event  adcstartEventB=Counter equals to zero (CTR=Zero)  adcstartEventB_type2=Counter equals to zero (CTR=Zero)  intEn=off  intPrd=First event  intSel=Counter equals to zero (CTR=Zero)  intSel_type2=Counter equals to zero (CTR=Zero)  hrpe=off  enHRPWM=off  HRPWM_LoadMode=Counter equals to period (CTR=PRD)  HRPWM_CTLMode=Duty or Period control mode  HRPWM_EDGMode=Both edge  hrpeb=off  enHRPWMB=off  HRPWM_LoadModeB=Counter equals to zero (CTR=ZERO)  HRPWM_CTLModeB=Duty or Period control mode  HRPWM_EDGModeB=Both edge  enHRDBRED=off  enHRDBFED=off  enSFO=on  enautoconv=on  chopperEnable=off  chopperFrequency=1  chopperFirstwidth=1  chopperDuty=12.5%  tripZonesource=Specify via dialog  tzselOSHT1=on  tzselOSHT2=on  tzselOSHT3=off  tzselOSHT4=off  tzselOSHT5=off  tzselOSHT6=off  tzselOSHDCAEV1=off  tzselOSHDCBEV1=off  tzselCBC1=off  tzselCBC2=off  tzselCBC3=off  tzselCBC4=off  tzselCBC5=off  tzselCBC6=off  tzselCBCDCAEV2=off  tzselCBCDCBEV2=off  enTzOstIntr=off  enTzCbcIntr=off  enTzDCAEVT1Intr=off  enTzDCAEVT2Intr=off  enTzDCBEVT1Intr=off  enTzDCBEVT2Intr=off  tzclrCBCLatch=Counter equals to zero (CTR=Zero)  ePWMxAforced=Low  ePWMxBforced=Low  DCAEVT1forced=No action  DCBEVT1forced=No action  DCAEVT2forced=No action  DCBEVT2forced=No action  dcah=Trip Zone 1 input (TZ1)  dcal=Trip Zone 2 input (TZ2)  dcbh=Trip Zone 1 input (TZ1)  dcbl=Trip Zone 2 input (TZ2)  dcah_type2=GPTRIP1SEL/(TZ1)  dcal_type2=GPTRIP1SEL/(TZ1)  dcbh_type2=GPTRIP1SEL/(TZ1)  dcbl_type2=GPTRIP1SEL/(TZ1)  gendcaevt1=Event disabled  gendcaevt2=Event disabled  gendcbevt1=Event disabled  gendcbevt2=Event disabled  dcaevt1src=DCAEVT1 with sync  dcaevt2src=DCAEVT2 with sync  dcbevt1src=DCBEVT1 with sync  dcbevt2src=DCBEVT2 with sync  pulsesel=Counter equals to zero (CTR=Zero)  blankinv=off  blankoffset=0  blankwidth=0  evsrcsel=Filtered version of DCAEVT1 (DCAEVT1FILT)  encape=off
      settings: LibrarySourceBlock=c2838xlib/ePWM
  ePWM2 : c2802xlib/ePWM  PwmType=C2000_Type4_F2838x  useModule=ePWM2  ePWMxLINKTBPRD=Not Linked  periodUnits=Clock cycles  timerSource=Specify via dialog  timerPeriod_clk=PWM_Period  timerPeriod_sec=0.0001  tbshadow=Counter equals to zero  countingMode=Up-Down  phaseActiveEnable=Disable  phaseDirection=Count down after sync  phaseActive=0  synchronizationEnable=off  dcaevt1Sync=off  dcbevt1Sync=off  synchronizationOption=Disable  dcbevt1SyncOut=off  dcaevt1SyncOut=off  cmpdSyncOut=off  cmpcSyncOut=off  cmpbSyncOut=off  zeroSyncOut=off  swfSyncOut=off  perSynchronizationOption=Counter equals to period (CTR=PRD)  clockPrescale=1  HSclockPrescale=1  enswap=off  ePWMxAStatus=on  ePWMxAactionLogic1=Do nothing  ePWMxAactionLogic2=Do nothing  ePWMxAactionLogic3=Clear  ePWMxAactionLogic4=Set  ePWMxAactionLogic5=Do nothing  ePWMxAactionLogic6=Do nothing  ePWMxACSFenable=off  ePWMxACSFvalue=Forcing disable  ePWMxASFreload=Zero  ePWMxBStatus=on  ePWMxBactionLogic1=Set  ePWMxBactionLogic2=Clear  ePWMxBactionLogic3=Do nothing  ePWMxBactionLogic4=Do nothing  ePWMxBactionLogic5=Clear  ePWMxBactionLogic6=Set  ePWMxBCSFenable=off  ePWMxBCSFvalue=Forcing disable  ePWMxBSFreload=Zero  ePWNxBOutWay=off  ePWMxLINKCMPA=Not Linked  CMPAUnits=Clock cycles  CMPASource=Input port  CMPAValue_per=50  CMPAValue_clk=32000  enCMPAshadow=Counter equals to zero (CTR=Zero)  ePWMxLINKCMPB=Not Linked  CMPBUnits=Clock cycles  CMPBSource=Specify via dialog  CMPBValue_per=50  CMPBValue_clk=32000  enCMPBshadow=Counter equals to zero (CTR=Zero)  ePWMxLINKCMPC=Not Linked  CMPCUnits=Clock cycles  CMPCSource=Specify via dialog  CMPCValue_per=50  CMPCValue_clk=32000  enCMPCshadow=Counter equals to zero (CTR=Zero)  ePWMxLINKCMPD=Not Linked  CMPDUnits=Clock cycles  CMPDSource=Specify via dialog  CMPDValue_per=50  CMPDValue_clk=32000  enCMPDshadow=Counter equals to zero (CTR=Zero)  enableDBePWMxA=on  enableDBePWMxB=on  enhalfcycle=off  DBpolarity=Active high complementary (AHC)  DBedgeDelay=Positive  DBSource_ePWMxA=ePWMxA  DBSource_ePWMxB=ePWMxA  DBPeriodUnits=Clock cycles  DBperiodSource=Specify via dialog  REDperiod=PWM_DeadTime_Count  FEDperiod=PWM_DeadTime_Count  REDperiod_sec=0  FEDperiod_sec=0  LoadModeDBRED=Immediate without using shadow  LoadModeDBFED=Immediate without using shadow  adcstartModuleA=off  adcrequestEventA=First event  adcstartEventA=Digital Compare Module A Event 1 start of conversion (DCAEVT1.soc)  adcstartEventA_type2=Counter equals to zero (CTR=Zero)  adcstartModuleB=off  adcrequestEventB=First event  adcstartEventB=Counter equals to zero (CTR=Zero)  adcstartEventB_type2=Counter equals to zero (CTR=Zero)  intEn=off  intPrd=First event  intSel=Counter equals to zero (CTR=Zero)  intSel_type2=Counter equals to zero (CTR=Zero)  hrpe=off  enHRPWM=off  HRPWM_LoadMode=Counter equals to period (CTR=PRD)  HRPWM_CTLMode=Duty or Period control mode  HRPWM_EDGMode=Both edge  hrpeb=off  enHRPWMB=off  HRPWM_LoadModeB=Counter equals to zero (CTR=ZERO)  HRPWM_CTLModeB=Duty or Period control mode  HRPWM_EDGModeB=Both edge  enHRDBRED=off  enHRDBFED=off  enSFO=on  enautoconv=on  chopperEnable=off  chopperFrequency=1  chopperFirstwidth=1  chopperDuty=12.5%  tripZonesource=Specify via dialog  tzselOSHT1=on  tzselOSHT2=on  tzselOSHT3=off  tzselOSHT4=off  tzselOSHT5=off  tzselOSHT6=off  tzselOSHDCAEV1=off  tzselOSHDCBEV1=off  tzselCBC1=off  tzselCBC2=off  tzselCBC3=off  tzselCBC4=off  tzselCBC5=off  tzselCBC6=off  tzselCBCDCAEV2=off  tzselCBCDCBEV2=off  enTzOstIntr=off  enTzCbcIntr=off  enTzDCAEVT1Intr=off  enTzDCAEVT2Intr=off  enTzDCBEVT1Intr=off  enTzDCBEVT2Intr=off  tzclrCBCLatch=Counter equals to zero (CTR=Zero)  ePWMxAforced=Low  ePWMxBforced=Low  DCAEVT1forced=No action  DCBEVT1forced=No action  DCAEVT2forced=No action  DCBEVT2forced=No action  dcah=Trip Zone 1 input (TZ1)  dcal=Trip Zone 2 input (TZ2)  dcbh=Trip Zone 1 input (TZ1)  dcbl=Trip Zone 2 input (TZ2)  dcah_type2=GPTRIP1SEL/(TZ1)  dcal_type2=GPTRIP1SEL/(TZ1)  dcbh_type2=GPTRIP1SEL/(TZ1)  dcbl_type2=GPTRIP1SEL/(TZ1)  gendcaevt1=Event disabled  gendcaevt2=Event disabled  gendcbevt1=Event disabled  gendcbevt2=Event disabled  dcaevt1src=DCAEVT1 with sync  dcaevt2src=DCAEVT2 with sync  dcbevt1src=DCBEVT1 with sync  dcbevt2src=DCBEVT2 with sync  pulsesel=Counter equals to zero (CTR=Zero)  blankinv=off  blankoffset=0  blankwidth=0  evsrcsel=Filtered version of DCAEVT1 (DCAEVT1FILT)  encape=off
      settings: LibrarySourceBlock=c2838xlib/ePWM
  ePWM3 : c2802xlib/ePWM  PwmType=C2000_Type4_F2838x  useModule=ePWM3  ePWMxLINKTBPRD=Not Linked  periodUnits=Clock cycles  timerSource=Specify via dialog  timerPeriod_clk=PWM_Period  timerPeriod_sec=0.0001  tbshadow=Counter equals to zero  countingMode=Up-Down  phaseActiveEnable=Disable  phaseDirection=Count down after sync  phaseActive=0  synchronizationEnable=off  dcaevt1Sync=off  dcbevt1Sync=off  synchronizationOption=Disable  dcbevt1SyncOut=off  dcaevt1SyncOut=off  cmpdSyncOut=off  cmpcSyncOut=off  cmpbSyncOut=off  zeroSyncOut=off  swfSyncOut=off  perSynchronizationOption=Counter equals to period (CTR=PRD)  clockPrescale=1  HSclockPrescale=1  enswap=off  ePWMxAStatus=on  ePWMxAactionLogic1=Do nothing  ePWMxAactionLogic2=Do nothing  ePWMxAactionLogic3=Clear  ePWMxAactionLogic4=Set  ePWMxAactionLogic5=Do nothing  ePWMxAactionLogic6=Do nothing  ePWMxACSFenable=off  ePWMxACSFvalue=Forcing disable  ePWMxASFreload=Zero  ePWMxBStatus=on  ePWMxBactionLogic1=Set  ePWMxBactionLogic2=Clear  ePWMxBactionLogic3=Do nothing  ePWMxBactionLogic4=Do nothing  ePWMxBactionLogic5=Clear  ePWMxBactionLogic6=Set  ePWMxBCSFenable=off  ePWMxBCSFvalue=Forcing disable  ePWMxBSFreload=Zero  ePWNxBOutWay=off  ePWMxLINKCMPA=Not Linked  CMPAUnits=Clock cycles  CMPASource=Input port  CMPAValue_per=50  CMPAValue_clk=32000  enCMPAshadow=Counter equals to zero (CTR=Zero)  ePWMxLINKCMPB=Not Linked  CMPBUnits=Clock cycles  CMPBSource=Specify via dialog  CMPBValue_per=50  CMPBValue_clk=32000  enCMPBshadow=Counter equals to zero (CTR=Zero)  ePWMxLINKCMPC=Not Linked  CMPCUnits=Clock cycles  CMPCSource=Specify via dialog  CMPCValue_per=50  CMPCValue_clk=32000  enCMPCshadow=Counter equals to zero (CTR=Zero)  ePWMxLINKCMPD=Not Linked  CMPDUnits=Clock cycles  CMPDSource=Specify via dialog  CMPDValue_per=50  CMPDValue_clk=32000  enCMPDshadow=Counter equals to zero (CTR=Zero)  enableDBePWMxA=on  enableDBePWMxB=on  enhalfcycle=off  DBpolarity=Active high complementary (AHC)  DBedgeDelay=Positive  DBSource_ePWMxA=ePWMxA  DBSource_ePWMxB=ePWMxA  DBPeriodUnits=Clock cycles  DBperiodSource=Specify via dialog  REDperiod=PWM_DeadTime_Count  FEDperiod=PWM_DeadTime_Count  REDperiod_sec=0  FEDperiod_sec=0  LoadModeDBRED=Immediate without using shadow  LoadModeDBFED=Immediate without using shadow  adcstartModuleA=off  adcrequestEventA=First event  adcstartEventA=Digital Compare Module A Event 1 start of conversion (DCAEVT1.soc)  adcstartEventA_type2=Counter equals to zero (CTR=Zero)  adcstartModuleB=off  adcrequestEventB=First event  adcstartEventB=Counter equals to zero (CTR=Zero)  adcstartEventB_type2=Counter equals to zero (CTR=Zero)  intEn=off  intPrd=First event  intSel=Counter equals to zero (CTR=Zero)  intSel_type2=Counter equals to zero (CTR=Zero)  hrpe=off  enHRPWM=off  HRPWM_LoadMode=Counter equals to period (CTR=PRD)  HRPWM_CTLMode=Duty or Period control mode  HRPWM_EDGMode=Both edge  hrpeb=off  enHRPWMB=off  HRPWM_LoadModeB=Counter equals to zero (CTR=ZERO)  HRPWM_CTLModeB=Duty or Period control mode  HRPWM_EDGModeB=Both edge  enHRDBRED=off  enHRDBFED=off  enSFO=on  enautoconv=on  chopperEnable=off  chopperFrequency=1  chopperFirstwidth=1  chopperDuty=12.5%  tripZonesource=Specify via dialog  tzselOSHT1=on  tzselOSHT2=on  tzselOSHT3=off  tzselOSHT4=off  tzselOSHT5=off  tzselOSHT6=off  tzselOSHDCAEV1=off  tzselOSHDCBEV1=off  tzselCBC1=off  tzselCBC2=off  tzselCBC3=off  tzselCBC4=off  tzselCBC5=off  tzselCBC6=off  tzselCBCDCAEV2=off  tzselCBCDCBEV2=off  enTzOstIntr=off  enTzCbcIntr=off  enTzDCAEVT1Intr=off  enTzDCAEVT2Intr=off  enTzDCBEVT1Intr=off  enTzDCBEVT2Intr=off  tzclrCBCLatch=Counter equals to zero (CTR=Zero)  ePWMxAforced=Low  ePWMxBforced=Low  DCAEVT1forced=No action  DCBEVT1forced=No action  DCAEVT2forced=No action  DCBEVT2forced=No action  dcah=Trip Zone 1 input (TZ1)  dcal=Trip Zone 2 input (TZ2)  dcbh=Trip Zone 1 input (TZ1)  dcbl=Trip Zone 2 input (TZ2)  dcah_type2=GPTRIP1SEL/(TZ1)  dcal_type2=GPTRIP1SEL/(TZ1)  dcbh_type2=GPTRIP1SEL/(TZ1)  dcbl_type2=GPTRIP1SEL/(TZ1)  gendcaevt1=Event disabled  gendcaevt2=Event disabled  gendcbevt1=Event disabled  gendcbevt2=Event disabled  dcaevt1src=DCAEVT1 with sync  dcaevt2src=DCAEVT2 with sync  dcbevt1src=DCBEVT1 with sync  dcbevt2src=DCBEVT2 with sync  pulsesel=Counter equals to zero (CTR=Zero)  blankinv=off  blankoffset=0  blankwidth=0  evsrcsel=Filtered version of DCAEVT1 (DCAEVT1FILT)  encape=off
      settings: LibrarySourceBlock=c2838xlib/ePWM
  id : Subsystem  TreatAsAtomicUnit=on  RTWFcnName=Id_Fun
      settings: RTWFcnNameOpts=User specified
  iq : Subsystem  TreatAsAtomicUnit=on  RTWFcnName=Iq_Fun
      settings: RTWFcnNameOpts=User specified
  obs_id : Outport
  obs_iq : Outport  Port=2
  wires:
  Inverse Park Transform/1 -> SVPWMG/1(Valpha)
  Inverse Park Transform/2 -> SVPWMG/2(Vbeta)
  Park Transform/2 -> [iq], obs_iq/1  "obs_iq"
  Park Transform/1 -> [id], obs_id/1  "obs_id"
  [iq] -> iq/3(iq)
  [iq] -> id/3(iq)
  [id] -> iq/2(id)
  [id] -> id/2(id)
  iq_ref/1 -> [Iq_ref]
  ia/1 -> Clack/1(ia)
  ic/1 -> Clack/3(ic)
  ib/1 -> Clack/2(ib)
  [etheta] -> Park Transform/3
  id/1(ud_raw) -> [ud_raw]
  iq/1(uq_raw) -> [uq_raw]
  dq_voltage_limiter/1(ud_lim) -> [ud_lim]
  dq_voltage_limiter/2(uq_lim) -> [uq_lim]
  dq_voltage_limiter/3(du_d_z) -> [du_d_z]
  dq_voltage_limiter/4(du_q_z) -> [du_q_z]
  [ud_raw] -> dq_voltage_limiter/1(ud_raw)
  [du_d_z] -> id/5(du_d_z)
  [du_q_z] -> iq/5(du_q_z)
  Uq_Zero_EN/1 -> Switch2/2
  Constant1/1 -> Switch2/1
  [uq_raw] -> Switch2/3
  Switch2/1 -> dq_voltage_limiter/2(uq_raw)
  [Iq_ref] -> iq/1(Iq_ref)
  dq_voltage_limiter/5(sat_flag_z) -> [sat_flag_z]
  [Id_Ref] -> id/1(id_ref)
  Id_Ref/1 -> [Id_Ref]
  etheta/1 -> [etheta]
  [etheta] -> Inverse Park Transform/3
  we/1 -> [we]
  Uq_Zero_EN1/1 -> iq/6(uq_zero_en)
  Clack/2(ibeta) -> Park Transform/2
  Clack/1(ialpha) -> Park Transform/1
  SVPWMG/1(Duty_A) -> ePWM1/1
  SVPWMG/2(Duty_B) -> ePWM2/1
  SVPWMG/3(Duty_C) -> ePWM3/1
  [uq_lim] -> Inverse Park Transform/2
  [ud_lim] -> Inverse Park Transform/1
  [we] -> id/4(we)
  [we] -> iq/4(we)

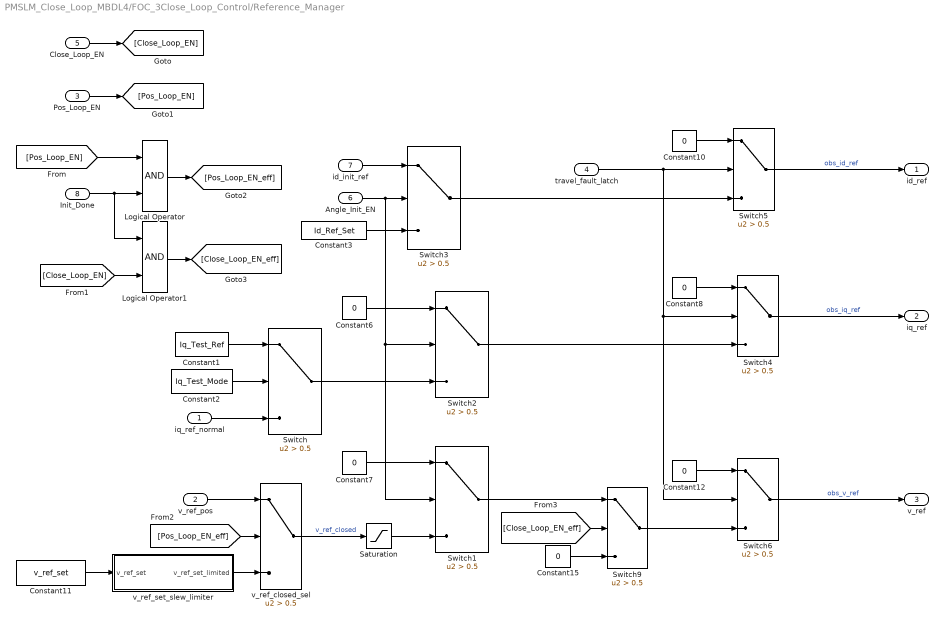
== system PMSLM_Close_Loop_MBDL4/FOC_3Close_Loop_Control/Reference_Manager ==
  iq_ref_normal : Inport
  v_ref_pos : Inport  Port=2
  Pos_Loop_EN : Inport  Port=3
  travel_fault_latch : Inport  Port=4
  Close_Loop_EN : Inport  Port=5
  Angle_Init_EN : Inport  Port=6
  id_init_ref : Inport  Port=7
  Init_Done : Inport  Port=8
  Constant1 : Constant  Value=Iq_Test_Ref
  Constant{6..8,10,12,15} (6 alike) : Constant  Value=0
  Constant11 : Constant  Value=v_ref_set  SampleTime=-1
  Constant2 : Constant  Value=Iq_Test_Mode
  Constant3 : Constant  Value=Id_Ref_Set
  Logical Operator : Logic  AllPortsSameDT=off  OutDataTypeStr=boolean
  Logical Operator1 : Logic  AllPortsSameDT=off  OutDataTypeStr=boolean
  Saturation : Saturate  UpperLimit=v_ref_max  LowerLimit=-v_ref_max
  Switch{,1..6,9} (8 alike) : Switch  Criteria=u2 > Threshold  Threshold=0.5  SaturateOnIntegerOverflow=off  InputSameDT=off
  v_ref_closed_sel : Switch  Criteria=u2 > Threshold  Threshold=0.5  SaturateOnIntegerOverflow=off  InputSameDT=off
  v_ref_set_slew_limiter : Subsystem
  id_ref : Outport
  iq_ref : Outport  Port=2
  v_ref : Outport  Port=3
  wires:
  Constant2/1 -> Switch/2
  Constant1/1 -> Switch/1
  iq_ref_normal/1 -> Switch/3
  v_ref_pos/1 -> v_ref_closed_sel/1
  v_ref_set_slew_limiter/1(v_ref_set_limited) -> v_ref_closed_sel/3
  v_ref_closed_sel/1 -> Saturation/1  "v_ref_closed"
  Constant7/1 -> Switch1/1
  Constant6/1 -> Switch2/1
  Switch/1 -> Switch2/3
  Switch2/1 -> Switch4/3
  Constant8/1 -> Switch4/1
  Constant10/1 -> Switch5/1
  travel_fault_latch/1 -> Switch5/2, Switch4/2, Switch6/2
  Constant11/1 -> v_ref_set_slew_limiter/1(v_ref_set)
  Constant12/1 -> Switch6/1
  Saturation/1 -> Switch1/3
  Close_Loop_EN/1 -> [Close_Loop_EN]
  Switch5/1 -> id_ref/1  "obs_id_ref"
  Switch4/1 -> iq_ref/1  "obs_iq_ref"
  Angle_Init_EN/1 -> Switch3/2, Switch2/2, Switch1/2
  id_init_ref/1 -> Switch3/1
  Constant3/1 -> Switch3/3
  Switch3/1 -> Switch5/3
  Switch6/1 -> v_ref/1  "obs_v_ref"
  Constant15/1 -> Switch9/3
  [Close_Loop_EN_eff] -> Switch9/2
  Switch9/1 -> Switch6/3
  Switch1/1 -> Switch9/1
  Pos_Loop_EN/1 -> [Pos_Loop_EN]
  [Pos_Loop_EN] -> Logical Operator/1
  Init_Done/1 -> Logical Operator1/1, Logical Operator/2
  Logical Operator/1 -> [Pos_Loop_EN_eff]
  [Close_Loop_EN] -> Logical Operator1/2
  Logical Operator1/1 -> [Close_Loop_EN_eff]
  [Pos_Loop_EN_eff] -> v_ref_closed_sel/2

== system PMSLM_Close_Loop_MBDL4/FOC_3Close_Loop_Control/Scheduler_10k_1k_100 ==
  note: 串口计数链(/10)
  note: position 计数链(/100)
  note: speed 计数链(/10)
  Add1 : Sum
  Add2 : Sum
  Add3 : Sum
  Constant1 : Constant
  Constant2 : Constant  Value=0
  Constant3 : Constant
  Constant4 : Constant  Value=0
  Constant5 : Constant
  Constant6 : Constant  Value=0
  Logical Operator : Logic  AllPortsSameDT=off  OutDataTypeStr=boolean
  UART_cnt_next_sel : Switch  Criteria=u2 > Threshold  Threshold=0.5  SaturateOnIntegerOverflow=off  InputSameDT=off
  UART_cnt_z : UnitDelay  SampleTime=-1
  UART_tc : simulink/Logic and Bit Operations/Compare To Constant  relop=>=  const=10  OutDataTypeStr=boolean
  pos_cnt_hold_sel : Switch  Criteria=u2 > Threshold  Threshold=0.5  SaturateOnIntegerOverflow=off  InputSameDT=off
  pos_cnt_update_sel : Switch  Criteria=u2 > Threshold  Threshold=0.5  SaturateOnIntegerOverflow=off  InputSameDT=off
  pos_cnt_z : UnitDelay  SampleTime=-1
  pos_tc : simulink/Logic and Bit Operations/Compare To Constant  relop=>=  const=10  OutDataTypeStr=boolean
  spd_cnt_next_sel : Switch  Criteria=u2 > Threshold  Threshold=0.5  SaturateOnIntegerOverflow=off  InputSameDT=off
  spd_cnt_z : UnitDelay  SampleTime=-1
  spd_tc : simulink/Logic and Bit Operations/Compare To Constant  relop=>=  const=10  OutDataTypeStr=boolean
  UART_tick : Outport
  speed_tick : Outport  Port=2
  pos_tick : Outport  Port=3
  wires:
  spd_cnt_z/1 -> [spd_cnt_z], Add1/1
  spd_tc/1 -> speed_tick/1, Logical Operator/1, pos_cnt_hold_sel/2, spd_cnt_next_sel/2
  Constant1/1 -> Add1/2
  Constant2/1 -> spd_cnt_next_sel/1
  spd_cnt_next_sel/1 -> spd_cnt_z/1
  Add1/1 -> spd_cnt_next_sel/3, spd_tc/1  "spd_cnt_inc"
  pos_cnt_z/1 -> Add2/1, pos_cnt_hold_sel/3
  Constant3/1 -> Add2/2
  Add2/1 -> pos_cnt_update_sel/3, pos_tc/1  "pos_cnt_inc"
  pos_tc/1 -> Logical Operator/2, pos_cnt_update_sel/2
  Constant4/1 -> pos_cnt_update_sel/1
  pos_cnt_update_sel/1 -> pos_cnt_hold_sel/1  "pos_cnt_update_candidate"
  pos_cnt_hold_sel/1 -> pos_cnt_z/1
  Logical Operator/1 -> pos_tick/1
  Constant6/1 -> UART_cnt_next_sel/1
  UART_tc/1 -> UART_tick/1, UART_cnt_next_sel/2
  UART_cnt_next_sel/1 -> UART_cnt_z/1
  Add3/1 -> UART_cnt_next_sel/3, UART_tc/1  "UART_cnt_inc"
  UART_cnt_z/1 -> Add3/1
  Constant5/1 -> Add3/2

== system PMSLM_Close_Loop_MBDL4/FOC_3Close_Loop_Control/Triggered_Position_loop ==
  x_ref_mm : Inport
  x_mm : Inport  Port=2
  pos_pi_reset : Inport  Port=3
  v_ff_pos : Inport  Port=4
  Trigger : TriggerPort  VariantControl=(inherit)
  Dead Zone : DeadZone  LowerValue=-Pos_deadband  UpperValue=+Pos_deadband
  Gain : Gain  Gain=Kp_pos
  Saturation : Saturate  UpperLimit=V_pos_max_mmps  LowerLimit=-V_pos_max_mmps
  Sum : Sum  Inputs=|+-
  Sum1 : Sum  Inputs=|++
  Terminator : Terminator
  v_ref_pos : Outport
  wires:
  x_ref_mm/1 -> Sum/1
  x_mm/1 -> Sum/2
  Sum/1 -> Dead Zone/1  "e_pos"
  Dead Zone/1 -> Gain/1
  Gain/1 -> Sum1/1
  v_ff_pos/1 -> Sum1/2
  Sum1/1 -> Saturation/1
  pos_pi_reset/1 -> Terminator/1
  Saturation/1 -> v_ref_pos/1  "obs_v_ref_pos"
